simulink model "testbench_encoder"  (R2015a)
settings: Solver=ode3  StartTime=0.0  StopTime=inf  RelTol=1e-3
libraries: legoev3lib x3
settings Model: SimulationMode=external  ExtModeTrigDuration=2  Creator=USER  LastModifiedBy=Keshav
settings OptimizationCC: OptimizeModelRefInitCode=on  LifeSpan=1
settings DebuggingCC: UnderspecifiedInitializationDetection=Classic  MergeDetectMultiDrivingBlocksExec=none
settings HardwareCC: ProdLargestAtomicInteger=Long  ProdLargestAtomicFloat=Float  ProdEndianess=LittleEndian  ProdHWDeviceType=ARM Compatible->ARM 9
settings RTWCC: SystemTargetFile=realtime.tlc  GenerateMakefile=off  TemplateMakefile=realtime.tmf  Description=Run on Target Hardware  RTWVerbose=off
settings ERTTargetCC: CombineOutputUpdateFcns=off  ERTSrcFileBannerTemplate=realtime_code_template.cgt  ERTHdrFileBannerTemplate=realtime_code_template.cgt  ERTDataSrcFileTemplate=realtime_code_template.cgt  ERTDataHdrFileTemplate=realtime_code_template.cgt  ERTCustomFileTemplate=realtime_file_process.tlc

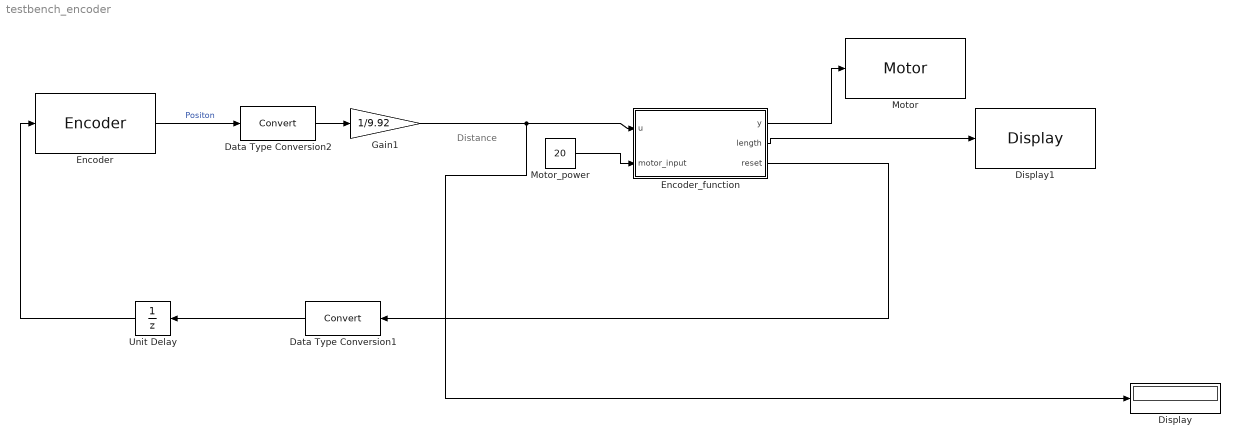
== system testbench_encoder ==
  note: Distance
  Data Type Conversion1 : DataTypeConversion
  Data Type Conversion2 : DataTypeConversion
  Display : Display
  Display1 : legoev3lib/Display  slcdLine=1  slcdFormat=Decimal
  Encoder : legoev3lib/Encoder  portNumber=A  opMode=Reset by external signal  sampleTime=0.1
  Encoder_function : MATLAB Function  TreatAsAtomicUnit=on
  Gain1 : Gain  Gain=1/9.92
  Motor : legoev3lib/Motor  sportNumber=A  sstopAction=Brake
  Motor_power : Constant  Value=20
  Unit Delay : UnitDelay  SampleTime=-1
  wires:
  Data Type Conversion2/1 -> Gain1/1
  Encoder/1 -> Data Type Conversion2/1  "Positon"
  Gain1/1 -> Display/1, Encoder_function/1(u)
  Encoder_function/1(y) -> Motor/1
  Motor_power/1 -> Encoder_function/2(motor_input)
  Encoder_function/2(length) -> Display1/1
  Unit Delay/1 -> Encoder/1
  Data Type Conversion1/1 -> Unit Delay/1
  Encoder_function/3(reset) -> Data Type Conversion1/1

== matlab function testbench_encoder/Encoder_function ==
  data: u input; y output; motor_input input; length output; reset output
function [y,length,reset] = fcn(u,motor_input)
%#codegen
state2=0;
if(u>=30)&&(u<=35)
    y=motor_input;
    length=u;
    state2=1;
    reset=1;
else
    y=0;
    length=u;
    reset=0;
end
end
